simulink model "paliotta"  (R2016a)
settings: Solver=FixedStepAuto  StartTime=0.0  StopTime=1000  FixedStep=0.05  RelTol=1e-3
libraries: simulink x2
settings Model: Creator=Staciej  LastModifiedBy=Staciej

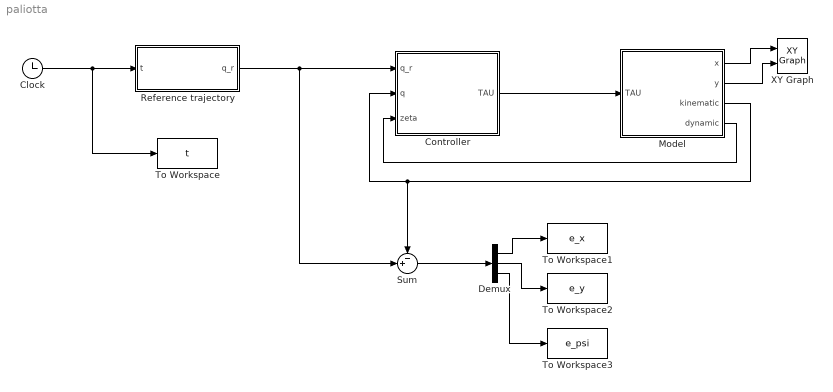
== system paliotta ==
  Clock : Clock
  Controller : Subsystem
  Demux : Demux  Outputs=3
  Model : Subsystem
  Reference trajectory : Subsystem
  Sum : Sum  Inputs=-+|
  To Workspace : ToWorkspace  VariableName=t  SampleTime=-1
  To Workspace1 : ToWorkspace  VariableName=e_x  SampleTime=-1
  To Workspace2 : ToWorkspace  VariableName=e_y  SampleTime=-1
  To Workspace3 : ToWorkspace  VariableName=e_psi  SampleTime=-1
  XY Graph : simulink/Sinks/XY Graph  xmin=-100  xmax=1000  ymin=-200  ymax=200  st=-1
  wires:
  Clock/1 -> To Workspace/1, Reference trajectory/1(t)
  Model/1(x) -> XY Graph/1
  Model/2(y) -> XY Graph/2
  Reference trajectory/1(q_r) -> Controller/1(q_r), Sum/2
  Model/4(dynamic) -> Controller/3(zeta)
  Model/3(kinematic) -> Controller/2(q), Sum/1
  Demux/1 -> To Workspace1/1
  Demux/2 -> To Workspace2/1
  Sum/1 -> Demux/1
  Controller/1(TAU) -> Model/1(TAU)
  Demux/3 -> To Workspace3/1

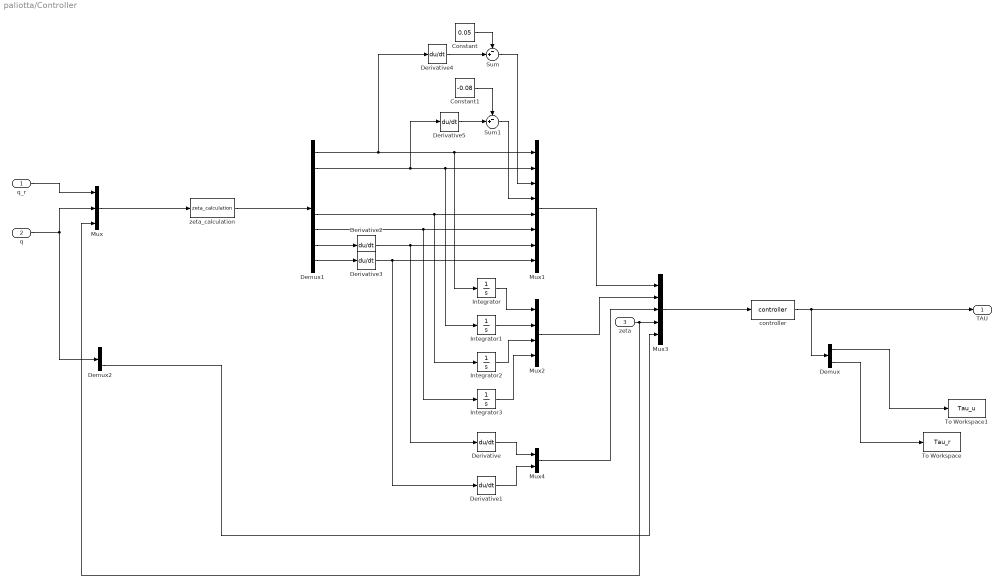
== system paliotta/Controller ==
  q_r : Inport
  q : Inport  Port=2
  zeta : Inport  Port=3
  Constant : Constant  Value=0.05
  Constant1 : Constant  Value=-0.08
  Demux : Demux  Outputs=2
  Demux1 : Demux  Outputs=8
  Demux2 : Demux  Outputs=3
  Derivative{,1..5} (6 alike) : Derivative
  Integrator{,1..3} (4 alike) : Integrator
  Mux : Mux  Inputs=3
  Mux1 : Mux  Inputs=8
  Mux2 : Mux
  Mux3 : Mux  Inputs=5
  Mux4 : Mux  Inputs=2
  Sum : Sum  Inputs=-+|
  Sum1 : Sum  Inputs=-+|
  To Workspace : ToWorkspace  VariableName=Tau_r  SampleTime=-1
  To Workspace1 : ToWorkspace  VariableName=Tau_u  SampleTime=-1
  controller : MATLABFcn  MATLABFcn=controller  OutputDimensions=2
  zeta_calculation : MATLABFcn  MATLABFcn=zeta_calculation  OutputDimensions=8
  TAU : Outport
  wires:
  controller/1 -> TAU/1, Demux/1
  q_r/1 -> Mux/1
  q/1 -> Demux2/1, Mux/2
  Mux/1 -> zeta_calculation/1
  zeta_calculation/1 -> Demux1/1
  Demux1/1 -> Derivative4/1, Integrator/1, Mux1/1
  Demux1/2 -> Derivative5/1, Integrator1/1, Mux1/2
  Demux1/5 -> Integrator2/1, Mux1/5
  Demux1/6 -> Integrator3/1, Mux1/6
  Demux1/7 -> Derivative2/1
  Demux1/8 -> Derivative3/1
  Integrator/1 -> Mux2/1
  Integrator1/1 -> Mux2/2
  Integrator2/1 -> Mux2/3
  Integrator3/1 -> Mux2/4
  Mux1/1 -> Mux3/1
  Mux2/1 -> Mux3/2
  Mux3/1 -> controller/1
  zeta/1 -> Mux/3, Mux3/4
  Demux2/3 -> Mux3/5
  Derivative1/1 -> Mux4/2
  Derivative/1 -> Mux4/1
  Mux4/1 -> Mux3/3
  Derivative2/1 -> Derivative/1, Mux1/7
  Derivative3/1 -> Derivative1/1, Mux1/8
  Constant/1 -> Sum/1
  Derivative4/1 -> Sum/2
  Derivative5/1 -> Sum1/2
  Constant1/1 -> Sum1/1
  Demux/1 -> To Workspace1/1
  Demux/2 -> To Workspace/1
  Sum/1 -> Mux1/3
  Sum1/1 -> Mux1/4

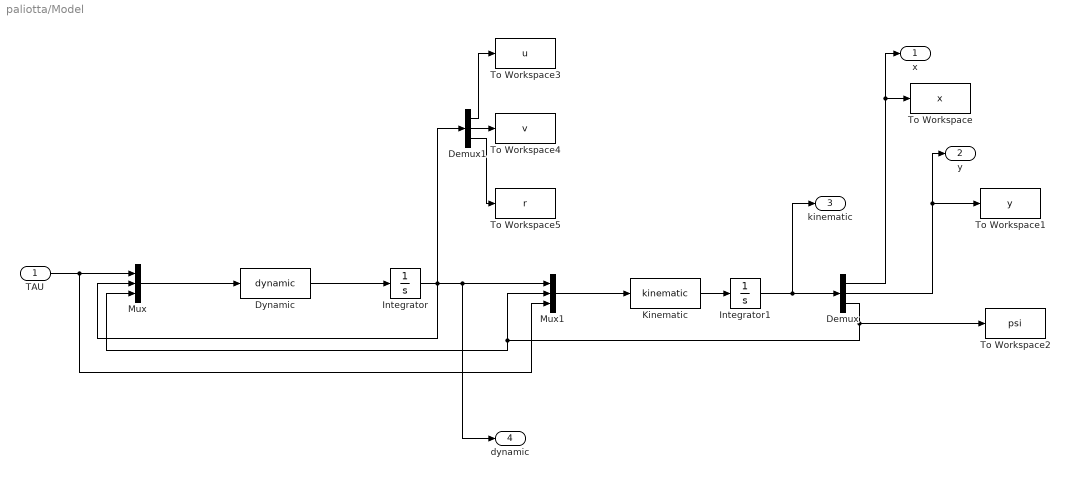
== system paliotta/Model ==
  TAU : Inport
  Demux : Demux  Outputs=3
  Demux1 : Demux  Outputs=3
  Dynamic : MATLABFcn  MATLABFcn=dynamic  OutputDimensions=3
  Integrator : Integrator  InitialCondition=[0 0 0]
  Integrator1 : Integrator  InitialCondition=[5 10 0]
  Kinematic : MATLABFcn  MATLABFcn=kinematic  OutputDimensions=3
  Mux : Mux  Inputs=3
  Mux1 : Mux  Inputs=3
  To Workspace : ToWorkspace  VariableName=x  SampleTime=-1
  To Workspace1 : ToWorkspace  VariableName=y  SampleTime=-1
  To Workspace2 : ToWorkspace  VariableName=psi  SampleTime=-1
  To Workspace3 : ToWorkspace  VariableName=u  SampleTime=-1
  To Workspace4 : ToWorkspace  VariableName=v  SampleTime=-1
  To Workspace5 : ToWorkspace  VariableName=r  SampleTime=-1
  x : Outport
  y : Outport  Port=2
  kinematic : Outport  Port=3
  dynamic : Outport  Port=4
  wires:
  TAU/1 -> Mux1/3, Mux/1
  Mux/1 -> Dynamic/1
  Dynamic/1 -> Integrator/1
  Integrator/1 -> Mux/2, Demux1/1, dynamic/1, Mux1/1
  Mux1/1 -> Kinematic/1
  Kinematic/1 -> Integrator1/1
  Demux/3 -> To Workspace2/1, Mux/3, Mux1/2
  Demux/1 -> x/1, To Workspace/1
  Demux/2 -> y/1, To Workspace1/1
  Integrator1/1 -> kinematic/1, Demux/1
  Demux1/1 -> To Workspace3/1
  Demux1/2 -> To Workspace4/1
  Demux1/3 -> To Workspace5/1

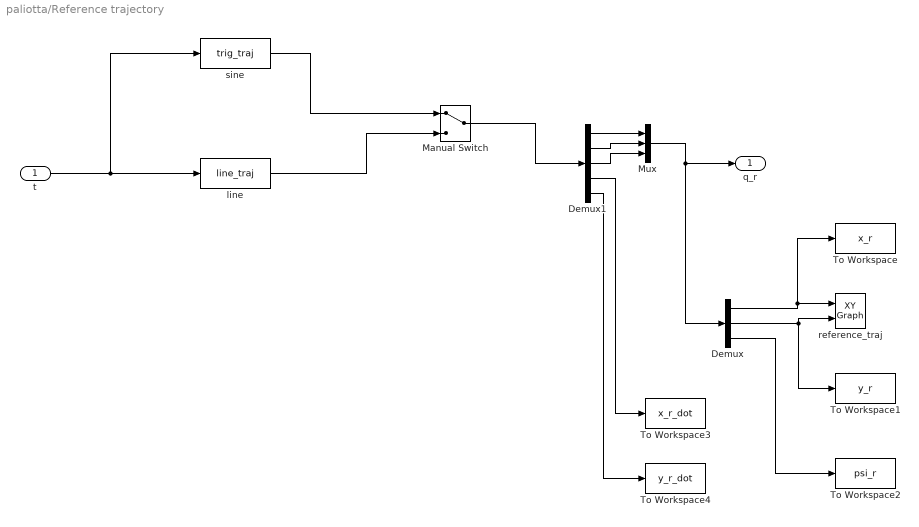
== system paliotta/Reference trajectory ==
  t : Inport
  Demux : Demux  Outputs=3
  Demux1 : Demux  Outputs=5
  Manual Switch : ManualSwitch
  Mux : Mux  Inputs=3
  To Workspace : ToWorkspace  VariableName=x_r  SampleTime=-1
  To Workspace1 : ToWorkspace  VariableName=y_r  SampleTime=-1
  To Workspace2 : ToWorkspace  VariableName=psi_r  SampleTime=-1
  To Workspace3 : ToWorkspace  VariableName=x_r_dot  SampleTime=-1
  To Workspace4 : ToWorkspace  VariableName=y_r_dot  SampleTime=-1
  line : MATLABFcn  MATLABFcn=line_traj  OutputDimensions=5
  reference_traj : simulink/Sinks/XY Graph  xmin=-100  xmax=1000  ymin=-200  ymax=200  st=-1
  sine : MATLABFcn  MATLABFcn=trig_traj  OutputDimensions=5
  q_r : Outport
  wires:
  t/1 -> sine/1, line/1
  Demux/1 -> To Workspace/1, reference_traj/1
  Demux/2 -> reference_traj/2, To Workspace1/1
  line/1 -> Manual Switch/2
  Demux/3 -> To Workspace2/1
  sine/1 -> Manual Switch/1
  Manual Switch/1 -> Demux1/1
  Demux1/1 -> Mux/1
  Demux1/2 -> Mux/2
  Demux1/3 -> Mux/3
  Mux/1 -> Demux/1, q_r/1
  Demux1/4 -> To Workspace3/1
  Demux1/5 -> To Workspace4/1
